simulink library "BLDC_Dynamics_lib"  (R2020a)
settings: Solver=VariableStepAuto  StartTime=0.0  StopTime=10.0  RelTol=1e-3
settings Model: Creator=enzoe  LastModifiedBy=enzoe

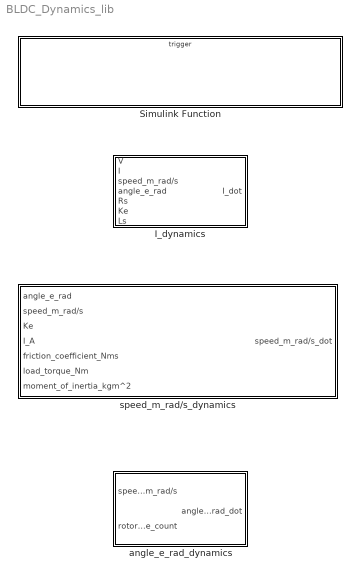
== system BLDC_Dynamics_lib ==
  I_dynamics : Subsystem
  Simulink Function : Subsystem  TreatAsAtomicUnit=on
  angle_e_rad_dynamics : Subsystem
  speed_m_rad/s_dynamics : Subsystem

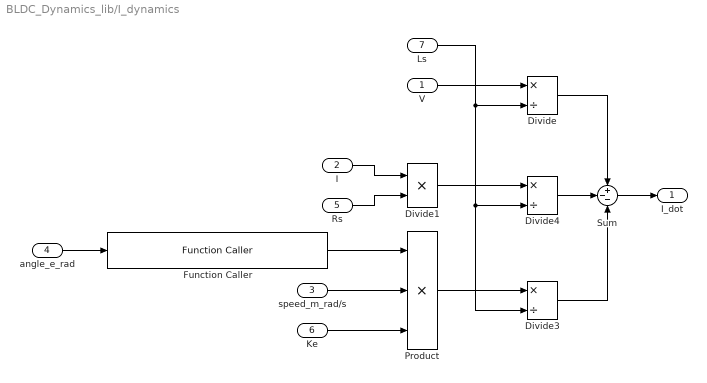
== system BLDC_Dynamics_lib/I_dynamics ==
  V : Inport
  I : Inport  Port=2
  speed_m_rad/s : Inport  Port=3
  angle_e_rad : Inport  Port=4
  Rs : Inport  Port=5
  Ke : Inport  Port=6
  Ls : Inport  Port=7
  Divide : Product  Inputs=*/
  Divide1 : Product  Inputs=**
  Divide3 : Product  Inputs=*/
  Divide4 : Product  Inputs=*/
  Function Caller : FunctionCaller  FunctionPrototype=BackEmf = BackEmfGenerator(angle_e_rad)  InputArgumentSpecifications=<Enter example>  OutputArgumentSpecifications=<Enter example>
  Product : Product  Inputs=3
  Sum : Sum  Inputs=+--
  I_dot : Outport
  wires:
  V/1 -> Divide/1
  I/1 -> Divide1/1
  Rs/1 -> Divide1/2
  angle_e_rad/1 -> Function Caller/1
  Ls/1 -> Divide3/2, Divide4/2, Divide/2
  Divide1/1 -> Divide4/1
  Divide/1 -> Sum/1
  Divide4/1 -> Sum/2
  Divide3/1 -> Sum/3
  Sum/1 -> I_dot/1
  Function Caller/1 -> Product/1
  speed_m_rad/s/1 -> Product/2
  Ke/1 -> Product/3
  Product/1 -> Divide3/1

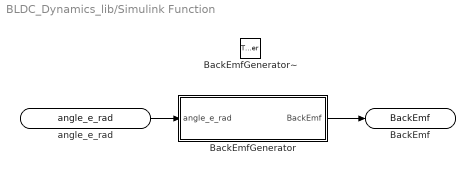
== system BLDC_Dynamics_lib/Simulink Function ==
  BackEmfGenerator~ : TriggerPort  TriggerType=function-call  IsSimulinkFunction=on  FunctionName=BackEmfGenerator  VariantControl=(inherit)
  BackEmfGenerator : MATLAB Function  TreatAsAtomicUnit=on
  angle_e_rad : ArgIn  DisableCoverage=on  ArgumentName=angle_e_rad
  BackEmf : ArgOut  DisableCoverage=on  ArgumentName=BackEmf
  wires:
  angle_e_rad/1 -> BackEmfGenerator/1(angle_e_rad)
  BackEmfGenerator/1(BackEmf) -> BackEmf/1

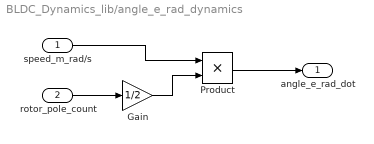
== system BLDC_Dynamics_lib/angle_e_rad_dynamics ==
  speed_m_rad/s : Inport
  rotor_pole_count : Inport  Port=2
  Gain : Gain  Gain=1/2
  Product : Product
  angle_e_rad_dot : Outport
  wires:
  rotor_pole_count/1 -> Gain/1
  Gain/1 -> Product/2
  speed_m_rad/s/1 -> Product/1
  Product/1 -> angle_e_rad_dot/1

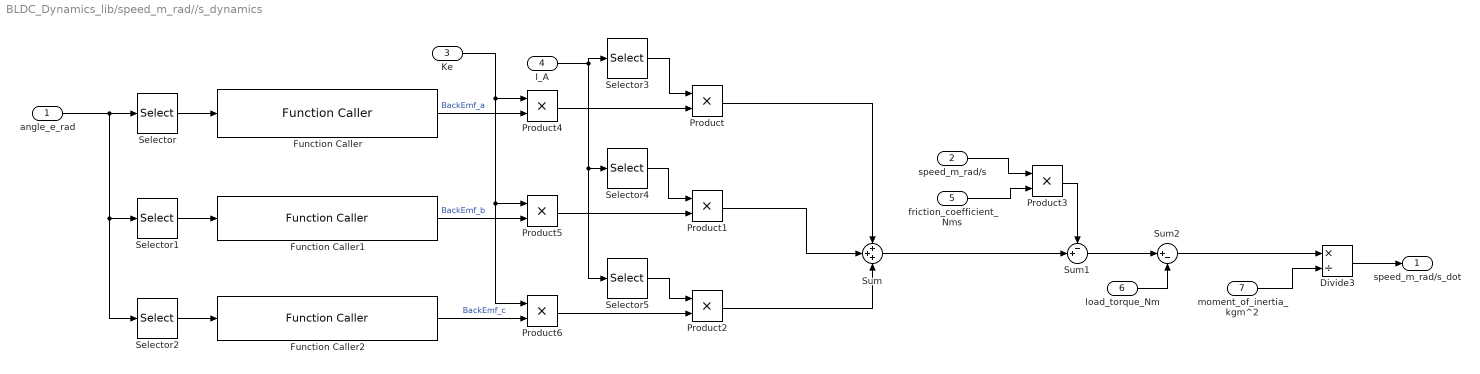
== system BLDC_Dynamics_lib/speed_m_rad//s_dynamics ==
  angle_e_rad : Inport
  speed_m_rad/s : Inport  Port=2
  Ke : Inport  Port=3
  I_A : Inport  Port=4
  friction_coefficient_Nms : Inport  Port=5
  load_torque_Nm : Inport  Port=6
  moment_of_inertia_kgm^2 : Inport  Port=7
  Divide3 : Product  Inputs=*/
  Function Caller : FunctionCaller  FunctionPrototype=BackEmf = BackEmfGenerator(angle_e_rad)  InputArgumentSpecifications=<Enter example>  OutputArgumentSpecifications=<Enter example>
  Function Caller1 : FunctionCaller  FunctionPrototype=BackEmf = BackEmfGenerator(angle_e_rad)  InputArgumentSpecifications=<Enter example>  OutputArgumentSpecifications=<Enter example>
  Function Caller2 : FunctionCaller  FunctionPrototype=BackEmf = BackEmfGenerator(angle_e_rad)  InputArgumentSpecifications=<Enter example>  OutputArgumentSpecifications=<Enter example>
  Product{,1..6} (7 alike) : Product
  Selector : Selector  InputPortWidth=3  IndexOptions=Index vector (dialog)  Indices=1  OutputSizes=1
  Selector1 : Selector  InputPortWidth=3  IndexOptions=Index vector (dialog)  Indices=2  OutputSizes=1
  Selector2 : Selector  InputPortWidth=3  IndexOptions=Index vector (dialog)  Indices=3  OutputSizes=1
  Selector3 : Selector  InputPortWidth=3  IndexOptions=Index vector (dialog)  Indices=1  OutputSizes=1
  Selector4 : Selector  InputPortWidth=3  IndexOptions=Index vector (dialog)  Indices=2  OutputSizes=1
  Selector5 : Selector  InputPortWidth=3  IndexOptions=Index vector (dialog)  Indices=3  OutputSizes=1
  Sum : Sum  Inputs=+++
  Sum1 : Sum  Inputs=-+|
  Sum2 : Sum  Inputs=|+-
  speed_m_rad/s_dot : Outport
  wires:
  speed_m_rad/s/1 -> Product3/1
  angle_e_rad/1 -> Selector2/1, Selector1/1, Selector/1
  Selector/1 -> Function Caller/1
  Selector2/1 -> Function Caller2/1
  Selector1/1 -> Function Caller1/1
  I_A/1 -> Selector3/1, Selector5/1, Selector4/1
  Selector3/1 -> Product/1
  Selector4/1 -> Product1/1
  Selector5/1 -> Product2/1
  Product1/1 -> Sum/2
  Product/1 -> Sum/1
  Product2/1 -> Sum/3
  friction_coefficient_Nms/1 -> Product3/2
  Sum1/1 -> Sum2/1
  load_torque_Nm/1 -> Sum2/2
  Sum2/1 -> Divide3/1
  moment_of_inertia_kgm^2/1 -> Divide3/2
  Divide3/1 -> speed_m_rad/s_dot/1
  Sum/1 -> Sum1/2
  Product3/1 -> Sum1/1
  Function Caller/1 -> Product4/2  "BackEmf_a"
  Function Caller1/1 -> Product5/2  "BackEmf_b"
  Function Caller2/1 -> Product6/2  "BackEmf_c"
  Ke/1 -> Product6/1, Product5/1, Product4/1
  Product4/1 -> Product/2
  Product5/1 -> Product1/2
  Product6/1 -> Product2/2

== matlab function BLDC_Dynamics_lib/Simulink Function/BackEmfGenerator ==
  data: angle_e_rad input; BackEmf output
function BackEmf = BackEmfGenerator(angle_e_rad)

% Generate the waveform
if (0 <= angle_e_rad && angle_e_rad < pi/6)
    BackEmf = angle_e_rad * 6/pi;
elseif (pi/6 <= angle_e_rad && angle_e_rad < 5*pi/6)
    BackEmf = 1;
elseif (5*pi/6 <= angle_e_rad && angle_e_rad < 7*pi/6)
    BackEmf = (pi - angle_e_rad) * 6/pi;
elseif (7*pi/6 <= angle_e_rad && angle_e_rad < 11*pi/6)
    BackEmf = -1;
elseif (11*pi/6 <= angle_e_rad && angle_e_rad < 2*pi)
    BackEmf = (angle_e_rad - 2*pi) * 6/pi;
else
    BackEmf = 0;
end

end
